simulink model "simu_red_atraso_adelanto"  (R2020a)
settings: Solver=VariableStepAuto  StartTime=0.0  StopTime=25  MaxStep=1e-3  RelTol=1e-3
values from neighbouring files (symbols this model uses):
  K = 1/div    [atraso_adelanto_c.m]
  p1 = p    [atraso_adelanto_c.m]
  p2 = 0.002    [atraso_adelanto_c.m]
  z1 = z    [atraso_adelanto_c.m]
  z2 = p2*razon    [atraso_adelanto_c.m]
libraries: simulink x1
settings Model: Creator=cmparedes  LastModifiedBy=cmparedes

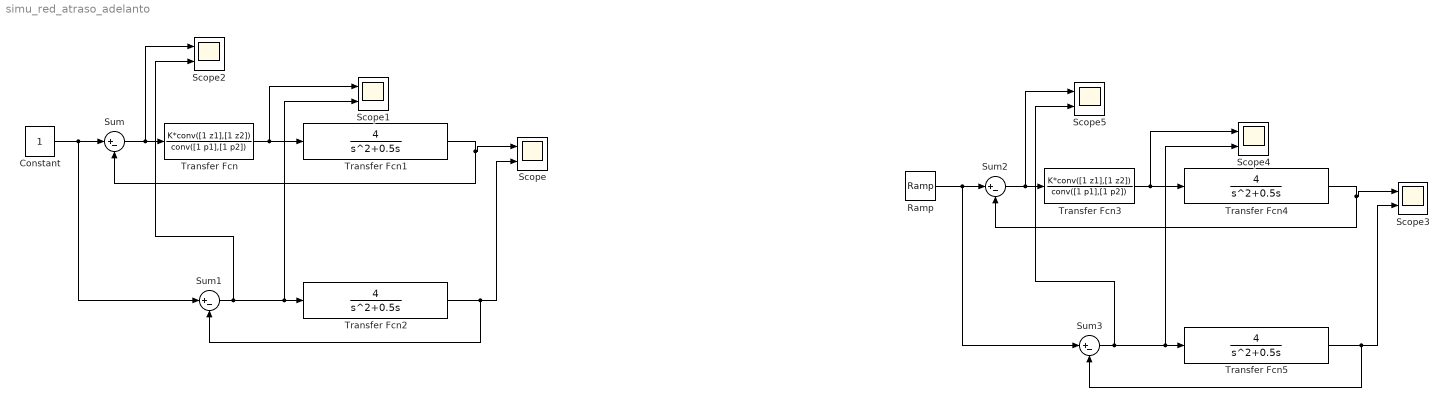
== system simu_red_atraso_adelanto ==
  Constant : Constant
  Ramp : simulink/Sources/Ramp  slope=1  start=0  InitialOutput=0
  Scope{,1..5} (6 alike) : Scope  NumInputPorts=2
  Sum{,1..3} (4 alike) : Sum  Inputs=|+-
  Transfer Fcn : TransferFcn  Numerator=K*conv([1 z1],[1 z2])  Denominator=conv([1 p1],[1 p2])
  Transfer Fcn{1..2,4..5} (4 alike) : TransferFcn  Numerator=4  Denominator=[1 0.5 0]
  Transfer Fcn3 : TransferFcn  Numerator=K*conv([1 z1],[1 z2])  Denominator=conv([1 p1],[1 p2])
  wires:
  Sum/1 -> Scope2/1, Transfer Fcn/1
  Transfer Fcn/1 -> Scope1/1, Transfer Fcn1/1
  Transfer Fcn1/1 -> Sum/2, Scope/1
  Constant/1 -> Sum1/1, Sum/1
  Sum1/1 -> Scope2/2, Transfer Fcn2/1, Scope1/2
  Transfer Fcn2/1 -> Scope/2, Sum1/2
  Ramp/1 -> Sum3/1, Sum2/1
  Transfer Fcn5/1 -> Scope3/2, Sum3/2
  Transfer Fcn4/1 -> Sum2/2, Scope3/1
  Sum2/1 -> Scope5/1, Transfer Fcn3/1
  Sum3/1 -> Scope5/2, Transfer Fcn5/1, Scope4/2
  Transfer Fcn3/1 -> Scope4/1, Transfer Fcn4/1
